simulink model "Model"  (R2020b)
settings: Solver=VariableStepAuto  StartTime=0.0  StopTime=20  MaxStep=0.1  RelTol=1e-1
values from neighbouring files (symbols this model uses):
  D = [0 ... (first row only)    [Data_clean.m]
  g = 9.81    [Data_clean.m]
  k_cart = 0.0113    [Data_clean.m]
  L = 5    [Data_clean.m]
  m = 12000    [Data_clean.m]
  M = 1000    [Data_clean.m]
  Ts = 0.1    [Data_clean.m]
undefined symbols (not defined in the file or in its folder): blk, Discrete, iA, isLTV, lastPcov, lastu, lastx, MDscale, mpc1_plant, MVscale, nCC, nu, nud, nv, nxp, ny, nym, p, RMVscale, Time, ts, uoff, X, xoff, Y, Yscale, Z
libraries: sm_lib x76, mpcsigdimcheck_private x76, nesl_utility x12, ctrlSharedLib x8, simulink_extras x5, mpclib x1
(part 3 of 8)

== system Model/3D3 ==
  X : Inport
  X_dot : Inport  Port=2
  Theta : Inport  Port=3
  Theta_dot : Inport  Port=4
  input2 : Inport  Port=5
  input1 : Inport  Port=6
  Brick Solid : sm_lib/Body Elements/Brick Solid  GraphicAmbientColor=[0.15 0.15 0.15 1.0]  BasedOnType=Mass  BrickDimensions=[15 3 0.5]  BrickDimensionUnits=m  CenterOfMass=[0 0 0]  CenterOfMassUnits=m  GraphicDiffuseColor=[0.5 0.5 0.5]  Density=1000  DensityUnits=kg/m^3  DoExposeReferenceFrame=on  GraphicEmissiveColor=[0.0 0.0 0.0 1.0]  ExportEntireGeometry=off  SerializedFrames=<Frames/>  MarkerShape=Sphere  MarkerSize=10  GraphicType=FromGeometry  InertiaType=CalculateFromGeometry  Mass=12500  MassUnits=kg  MomentsOfInertia=[1 1 1]  MomentsOfInertiaUnits=kg*m^2  GraphicOpacity=1.0  ProductsOfInertia=[0 0 0]  ProductsOfInertiaUnits=kg*m^2  GraphicShininess=75  GraphicSpecularColor=[0.5 0.5 0.5 1.0]  GraphicVisPropType=SimpleVisualProperties
      settings: SourceProductName=Multibody
  Brick Solid1 : sm_lib/Body Elements/Brick Solid  GraphicAmbientColor=[0.15 0.15 0.15 1.0]  BasedOnType=Mass  BrickDimensions=[2 2 0.5]  BrickDimensionUnits=m  CenterOfMass=[0 0 0]  CenterOfMassUnits=m  GraphicDiffuseColor=[1.0 0.2 0.2]  Density=1000  DensityUnits=kg/m^3  DoExposeReferenceFrame=on  GraphicEmissiveColor=[0.0 0.0 0.0 1.0]  ExportEntireGeometry=off  SerializedFrames=<Frames/>  MarkerShape=Sphere  MarkerSize=10  GraphicType=FromGeometry  InertiaType=CalculateFromGeometry  Mass=12500  MassUnits=kg  MomentsOfInertia=[1 1 1]  MomentsOfInertiaUnits=kg*m^2  GraphicOpacity=1.0  ProductsOfInertia=[0 0 0]  ProductsOfInertiaUnits=kg*m^2  GraphicShininess=75  GraphicSpecularColor=[0.5 0.5 0.5 1.0]  GraphicVisPropType=SimpleVisualProperties
      settings: SourceProductName=Multibody
  Cylindrical Solid : sm_lib/Body Elements/Cylindrical Solid  GraphicAmbientColor=[0.15 0.15 0.15 1.0]  BasedOnType=Density  CenterOfMass=[0 0 0]  CenterOfMassUnits=m  GraphicDiffuseColor=[1.0 0.8 0.0]  CylinderLength=L  CylinderLengthUnits=m  CylinderRadius=0.05  CylinderRadiusUnits=m  Density=1000  DensityUnits=kg/m^3  DoExposeReferenceFrame=on  GraphicEmissiveColor=[0.0 0.0 0.0 1.0]  ExportEntireGeometry=off  SerializedFrames=<Frames/>  MarkerShape=Sphere  MarkerSize=10  GraphicType=FromGeometry  InertiaType=CalculateFromGeometry  Mass=1  MassUnits=kg  MomentsOfInertia=[1 1 1]  MomentsOfInertiaUnits=kg*m^2  GraphicOpacity=1.0  ProductsOfInertia=[0 0 0]  ProductsOfInertiaUnits=kg*m^2  GraphicShininess=75  GraphicSpecularColor=[0.5 0.5 0.5 1.0]  GraphicVisPropType=SimpleVisualProperties
  Graphic : sm_lib/Body Elements/Graphic  Commented=on  GraphicType=Marker  MarkerShape=Frame  MarkerSize=20  GraphicVisPropType=SimpleVisualProperties  GraphicDiffuseColor=[0.6 0.6 1.0]  GraphicSpecularColor=[0.5 0.5 0.5 1.0]  GraphicAmbientColor=[0.15 0.15 0.15 1.0]  GraphicEmissiveColor=[0.0 0.0 0.0 1.0]  GraphicShininess=75  GraphicOpacity=1.0
  Graphic1 : sm_lib/Body Elements/Graphic  Commented=on  GraphicType=Marker  MarkerShape=Frame  MarkerSize=20  GraphicVisPropType=SimpleVisualProperties  GraphicDiffuseColor=[1.0 0.2 0.2]  GraphicSpecularColor=[0.5 0.5 0.5 1.0]  GraphicAmbientColor=[0.15 0.15 0.15 1.0]  GraphicEmissiveColor=[0.0 0.0 0.0 1.0]  GraphicShininess=75  GraphicOpacity=1.0
  Graphic2 : sm_lib/Body Elements/Graphic  Commented=on  GraphicType=Marker  MarkerShape=Frame  MarkerSize=20  GraphicVisPropType=SimpleVisualProperties  GraphicDiffuseColor=[0.8 0.8 0.0]  GraphicSpecularColor=[0.5 0.5 0.5 1.0]  GraphicAmbientColor=[0.15 0.15 0.15 1.0]  GraphicEmissiveColor=[0.0 0.0 0.0 1.0]  GraphicShininess=75  GraphicOpacity=1.0
  Graphic3 : sm_lib/Body Elements/Graphic  Commented=on  GraphicType=Marker  MarkerShape=Frame  MarkerSize=20  GraphicVisPropType=SimpleVisualProperties  GraphicDiffuseColor=[0.2 0.2 1.0]  GraphicSpecularColor=[0.5 0.5 0.5 1.0]  GraphicAmbientColor=[0.15 0.15 0.15 1.0]  GraphicEmissiveColor=[0.0 0.0 0.0 1.0]  GraphicShininess=75  GraphicOpacity=1.0
  Graphic4 : sm_lib/Body Elements/Graphic  Commented=on  GraphicType=Marker  MarkerShape=Frame  MarkerSize=20  GraphicVisPropType=SimpleVisualProperties  GraphicDiffuseColor=[0.8 1.0 0.0]  GraphicSpecularColor=[0.5 0.5 0.5 1.0]  GraphicAmbientColor=[0.15 0.15 0.15 1.0]  GraphicEmissiveColor=[0.0 0.0 0.0 1.0]  GraphicShininess=75  GraphicOpacity=1.0
  Mechanism Configuration : sm_lib/Utilities/Mechanism Configuration  UniformGravity=Constant  GravityVector=[0 0 -9.80665]  GravityVectorUnits=m/s^2  GravityUnits=m/s^2  LinearizationDelta=0.001  JointModeTransitionNonlinearIterations=2
      settings: SourceProductName=Multibody
  Prismatic Joint : sm_lib/Joints/Prismatic Joint  JointMode=Normal  SenseConstraintForce=off  SenseConstraintForceX=off  SenseConstraintForceY=off  SenseConstraintForceZ=off  SenseConstraintTorque=off  SenseConstraintTorqueX=off  SenseConstraintTorqueY=off  SenseConstraintTorqueZ=off  SenseTotalForce=off  SenseTotalForceX=off  SenseTotalForceY=off  SenseTotalForceZ=off  SenseTotalTorque=off  SenseTotalTorqueX=off  SenseTotalTorqueY=off  SenseTotalTorqueZ=off  CompositeWrenchDir=FollowerOnBase  CompositeWrenchFrame=BaseFrame  EquilibriumPosition=0  EquilibriumPositionUnits=m  SpringStiffness=0  SpringStiffnessUnits=N/m  DampingCoefficient=0  DampingCoefficientUnits=N/(m/s)  TorqueActuationMode=ComputedTorque  MotionActuationMode=InputMotion  SensePosition=off  SenseVelocity=off  SenseAcceleration=off  SenseTorqueForce=off  SenseLowerLimitTorqueForce=off  SenseUpperLimitTorqueForce=off  LowerLimitSpecify=off  LowerLimitBound=-1  LowerLimitBoundUnits=m  LowerLimitStiffness=1e6  LowerLimitStiffnessUnits=N/m  LowerLimitDamping=1e3  LowerLimitDampingUnits=N/(m/s)  LowerLimitTransitionRegionWidth=1e-4  LowerLimitTransitionRegionWidthUnits=m  UpperLimitSpecify=off  UpperLimitBound=1  UpperLimitBoundUnits=m  UpperLimitStiffness=1e6  UpperLimitStiffnessUnits=N/m  UpperLimitDamping=1e3  UpperLimitDampingUnits=N/(m/s)  UpperLimitTransitionRegionWidth=1e-4  UpperLimitTransitionRegionWidthUnits=m  PositionTargetSpecify=off  PositionTargetPriority=High  PositionTargetValue=0  PositionTargetValueUnits=m  VelocityTargetSpecify=off  VelocityTargetPriority=High  VelocityTargetValue=0  VelocityTargetValueUnits=m/s
  Revolute Joint : sm_lib/Joints/Revolute Joint  JointMode=Normal  SenseConstraintForce=off  SenseConstraintForceX=off  SenseConstraintForceY=off  SenseConstraintForceZ=off  SenseConstraintTorque=off  SenseConstraintTorqueX=off  SenseConstraintTorqueY=off  SenseConstraintTorqueZ=off  SenseTotalForce=off  SenseTotalForceX=off  SenseTotalForceY=off  SenseTotalForceZ=off  SenseTotalTorque=off  SenseTotalTorqueX=off  SenseTotalTorqueY=off  SenseTotalTorqueZ=off  CompositeWrenchDir=FollowerOnBase  CompositeWrenchFrame=BaseFrame  EquilibriumPosition=0  EquilibriumPositionUnits=deg  SpringStiffness=0  SpringStiffnessUnits=N*m/deg  DampingCoefficient=0  DampingCoefficientUnits=N*m/(deg/s)  TorqueActuationMode=ComputedTorque  MotionActuationMode=InputMotion  SensePosition=off  SenseVelocity=off  SenseAcceleration=off  SenseTorqueForce=off  SenseLowerLimitTorqueForce=off  SenseUpperLimitTorqueForce=off  LowerLimitSpecify=off  LowerLimitBound=-90  LowerLimitBoundUnits=deg  LowerLimitStiffness=1e4  LowerLimitStiffnessUnits=N*m/deg  LowerLimitDamping=10  LowerLimitDampingUnits=N*m/(deg/s)  LowerLimitTransitionRegionWidth=0.1  LowerLimitTransitionRegionWidthUnits=deg  UpperLimitSpecify=off  UpperLimitBound=90  UpperLimitBoundUnits=deg  UpperLimitStiffness=1e4  UpperLimitStiffnessUnits=N*m/deg  UpperLimitDamping=10  UpperLimitDampingUnits=N*m/(deg/s)  UpperLimitTransitionRegionWidth=0.1  UpperLimitTransitionRegionWidthUnits=deg  PositionTargetSpecify=off  PositionTargetPriority=High  PositionTargetValue=0.2  PositionTargetValueUnits=rad  VelocityTargetSpecify=off  VelocityTargetPriority=High  VelocityTargetValue=0  VelocityTargetValueUnits=deg/s
  Rigid Transform : sm_lib/Frames and Transforms/Rigid Transform  TranslationMethod=StandardAxis  TranslationStandardOffset=6.5  TranslationLengthUnit=m  TranslationStandardAxis=-X  TranslationCartesianOffset=[0 0 0]  TranslationROffset=0  TranslationROffsetUnits=m  TranslationZOffset=0  TranslationZOffsetUnits=m  TranslationThetaOffset=0  TranslationThetaOffsetUnits=deg  RotationMethod=None  RotationAngleUnits=deg  RotationStandardAxis=+Z  RotationAngle=0.0  RotationArbitraryAxis=[0 0 1]  FollAlignAxisA=+X  BaseAlignAxisA=+X  FollAlignAxisB=+Z  BaseAlignAxisB=-Z  RotationSequenceAxes=FollowerAxes  RotationSequence=XYX  RotationSequenceAngles=[0 0 0]  RotationSequenceAnglesUnits=deg  RotationMatrix=[1 0 0; 0 1 0; 0 0 1]
      settings: SourceProductName=Multibody
  Rigid Transform1 : sm_lib/Frames and Transforms/Rigid Transform  TranslationMethod=None  TranslationStandardOffset=0.5  TranslationLengthUnit=m  TranslationStandardAxis=+Z  TranslationCartesianOffset=[0 0 0]  TranslationROffset=0  TranslationROffsetUnits=m  TranslationZOffset=0  TranslationZOffsetUnits=m  TranslationThetaOffset=0  TranslationThetaOffsetUnits=deg  RotationMethod=AlignedAxes  RotationAngleUnits=deg  RotationStandardAxis=+Z  RotationAngle=0.0  RotationArbitraryAxis=[0 0 1]  FollAlignAxisA=+X  BaseAlignAxisA=+Z  FollAlignAxisB=+Y  BaseAlignAxisB=+Y  RotationSequenceAxes=FollowerAxes  RotationSequence=XYX  RotationSequenceAngles=[0 0 0]  RotationSequenceAnglesUnits=deg  RotationMatrix=[1 0 0; 0 1 0; 0 0 1]
      settings: SourceProductName=Multibody
  Rigid Transform2 : sm_lib/Frames and Transforms/Rigid Transform  TranslationMethod=StandardAxis  TranslationStandardOffset=0.5  TranslationLengthUnit=m  TranslationStandardAxis=+Z  TranslationCartesianOffset=[0 0 0]  TranslationROffset=0  TranslationROffsetUnits=m  TranslationZOffset=0  TranslationZOffsetUnits=m  TranslationThetaOffset=0  TranslationThetaOffsetUnits=deg  RotationMethod=AlignedAxes  RotationAngleUnits=deg  RotationStandardAxis=+Z  RotationAngle=0.0  RotationArbitraryAxis=[0 0 1]  FollAlignAxisA=+Z  BaseAlignAxisA=+X  FollAlignAxisB=+Y  BaseAlignAxisB=+Y  RotationSequenceAxes=FollowerAxes  RotationSequence=XYX  RotationSequenceAngles=[0 0 0]  RotationSequenceAnglesUnits=deg  RotationMatrix=[1 0 0; 0 1 0; 0 0 1]
      settings: SourceProductName=Multibody
  Rigid Transform3 : sm_lib/Frames and Transforms/Rigid Transform  TranslationMethod=StandardAxis  TranslationStandardOffset=L/2  TranslationLengthUnit=m  TranslationStandardAxis=-Z  TranslationCartesianOffset=[0 0 0]  TranslationROffset=0  TranslationROffsetUnits=m  TranslationZOffset=0  TranslationZOffsetUnits=m  TranslationThetaOffset=0  TranslationThetaOffsetUnits=deg  RotationMethod=None  RotationAngleUnits=deg  RotationStandardAxis=+Z  RotationAngle=0.0  RotationArbitraryAxis=[0 0 1]  FollAlignAxisA=+X  BaseAlignAxisA=+X  FollAlignAxisB=+Z  BaseAlignAxisB=+Y  RotationSequenceAxes=FollowerAxes  RotationSequence=XYX  RotationSequenceAngles=[0 0 0]  RotationSequenceAnglesUnits=deg  RotationMatrix=[1 0 0; 0 1 0; 0 0 1]
      settings: SourceProductName=Multibody
  Rigid Transform4 : sm_lib/Frames and Transforms/Rigid Transform  TranslationMethod=None  TranslationStandardOffset=2.5  TranslationLengthUnit=m  TranslationStandardAxis=-Z  TranslationCartesianOffset=[0 0 0]  TranslationROffset=0  TranslationROffsetUnits=m  TranslationZOffset=0  TranslationZOffsetUnits=m  TranslationThetaOffset=0  TranslationThetaOffsetUnits=deg  RotationMethod=AlignedAxes  RotationAngleUnits=deg  RotationStandardAxis=+Z  RotationAngle=0.0  RotationArbitraryAxis=[0 0 1]  FollAlignAxisA=+X  BaseAlignAxisA=+X  FollAlignAxisB=+Y  BaseAlignAxisB=+Z  RotationSequenceAxes=FollowerAxes  RotationSequence=XYX  RotationSequenceAngles=[0 0 0]  RotationSequenceAnglesUnits=deg  RotationMatrix=[1 0 0; 0 1 0; 0 0 1]
      settings: SourceProductName=Multibody
  Rigid Transform5 : sm_lib/Frames and Transforms/Rigid Transform  TranslationMethod=StandardAxis  TranslationStandardOffset=L/2  TranslationLengthUnit=m  TranslationStandardAxis=-Y  TranslationCartesianOffset=[0 0 0]  TranslationROffset=0  TranslationROffsetUnits=m  TranslationZOffset=0  TranslationZOffsetUnits=m  TranslationThetaOffset=0  TranslationThetaOffsetUnits=deg  RotationMethod=AlignedAxes  RotationAngleUnits=deg  RotationStandardAxis=+Z  RotationAngle=0.0  RotationArbitraryAxis=[0 0 1]  FollAlignAxisA=+X  BaseAlignAxisA=+X  FollAlignAxisB=+Z  BaseAlignAxisB=+Y  RotationSequenceAxes=FollowerAxes  RotationSequence=XYX  RotationSequenceAngles=[0 0 0]  RotationSequenceAnglesUnits=deg  RotationMatrix=[1 0 0; 0 1 0; 0 0 1]
      settings: SourceProductName=Multibody
  Simulink-PS Converter : nesl_utility/Simulink-PS Converter  PhysicalDomain=network_engine_domain  SubClassName=ps_input  LeftPortType=input  RightPortType=output  PseudoPeriodic=off  Frequencies=[]  NoiseDistribution=none  NoiseParameters=[]  Unit=1  AffineConversion=off  FilteringAndDerivatives=provide  SimscapeFilterOrder=1  InputFilterTimeConstant=0.001  UdotUserProvided=2
  Simulink-PS Converter1 : nesl_utility/Simulink-PS Converter  PhysicalDomain=network_engine_domain  SubClassName=ps_input  LeftPortType=input  RightPortType=output  PseudoPeriodic=off  Frequencies=[]  NoiseDistribution=none  NoiseParameters=[]  Unit=1  AffineConversion=off  FilteringAndDerivatives=provide  SimscapeFilterOrder=1  InputFilterTimeConstant=0.001  UdotUserProvided=2
  Solver Configuration : nesl_utility/Solver Configuration  PhysicalDomain=network_engine_domain  SubClassName=solver  LeftPortType=input  RightPortType=generic  Tones=[]  Harmonics=[]  SimulateNoise=off  Profile=off  UseLocalSampling=off  EnableSwitchedLinearOptims=on  FrequencyDomain=off  UseCCode=off  RelTol=0.001  AbsTol=1e-06  MinStep=1e-09  ToWorkspace=off  RevertToSquareIcSolve=off  NumHomotopyIterations=100  PhasorMode=off  PhasorModeNumHarmonics=1  DoDC=off  ResidualTolerance=1e-09  UseLocalSolver=off  LocalSolverChoice=NE_BACKWARD_EULER_ADVANCER  LocalSolverSampleTime=0.001  DoFixedCost=off  MaxNonlinIter=3  MaxModeIter=2  ComputeImpulses=off  ImpulseIterations=2  LinearAlgebra=Sparse  EquationFormulation=NE_TIME_EF  DelaysMemoryBudget=1024  AutomaticFiltering=on  FilteringTimeConstant=0.001  PartitionStorageMethod=AS_NEEDED  PartitionMemoryBudget=1024  PartitionMethod=FAST
      settings: SourceProductName=Utilities
  Spherical Solid : sm_lib/Body Elements/Spherical Solid  GraphicAmbientColor=[0.15 0.15 0.15 1.0]  BasedOnType=Density  CenterOfMass=[0 0 0]  CenterOfMassUnits=m  GraphicDiffuseColor=[0.2 0.8 0.0]  Density=1000  DensityUnits=kg/m^3  DoExposeReferenceFrame=on  GraphicEmissiveColor=[0.0 0.0 0.0 1.0]  ExportEntireGeometry=off  SerializedExposedGeometries=<ExposedGeometries/>  SerializedFrames=<Frames/>  MarkerShape=Sphere  MarkerSize=10  GraphicType=FromGeometry  InertiaType=CalculateFromGeometry  Mass=1  MassUnits=kg  MomentsOfInertia=[1 1 1]  MomentsOfInertiaUnits=kg*m^2  GraphicOpacity=1.0  ProductsOfInertia=[0 0 0]  ProductsOfInertiaUnits=kg*m^2  GraphicShininess=75  GraphicSpecularColor=[0.5 0.5 0.5 1.0]  SphereRadius=0.5  SphereRadiusUnits=m  GraphicVisPropType=SimpleVisualProperties
  World Frame : sm_lib/Frames and Transforms/World Frame
      settings: SourceProductName=Multibody
  wires:
  Theta_dot/1 -> Simulink-PS Converter1/2
  input2/1 -> Simulink-PS Converter/3
  X/1 -> Simulink-PS Converter/1
  X_dot/1 -> Simulink-PS Converter/2
  Theta/1 -> Simulink-PS Converter1/1
  input1/1 -> Simulink-PS Converter1/3
  connections:
  Rigid Transform5/LConn1 -- Graphic3/RConn1 -- Revolute Joint/RConn1
  Rigid Transform3/LConn1 -- Rigid Transform5/RConn1 -- Cylindrical Solid/RConn1 -- Graphic4/RConn1
  Simulink-PS Converter1/RConn1 -- Revolute Joint/LConn2
  Rigid Transform4/LConn1 -- Brick Solid1/RConn1 -- Graphic2/RConn1 -- Rigid Transform1/RConn1
  Brick Solid/RConn1 -- Graphic/RConn1 -- World Frame/RConn1 -- Mechanism Configuration/RConn1 -- Solver Configuration/RConn1 -- Rigid Transform/LConn1
  Simulink-PS Converter/RConn1 -- Prismatic Joint/LConn2
  Rigid Transform1/LConn1 -- Prismatic Joint/RConn1
  Prismatic Joint/LConn1 -- Graphic1/RConn1 -- Rigid Transform2/RConn1
  Rigid Transform3/RConn1 -- Spherical Solid/RConn1
  Rigid Transform2/LConn1 -- Rigid Transform/RConn1
  Revolute Joint/LConn1 -- Rigid Transform4/RConn1

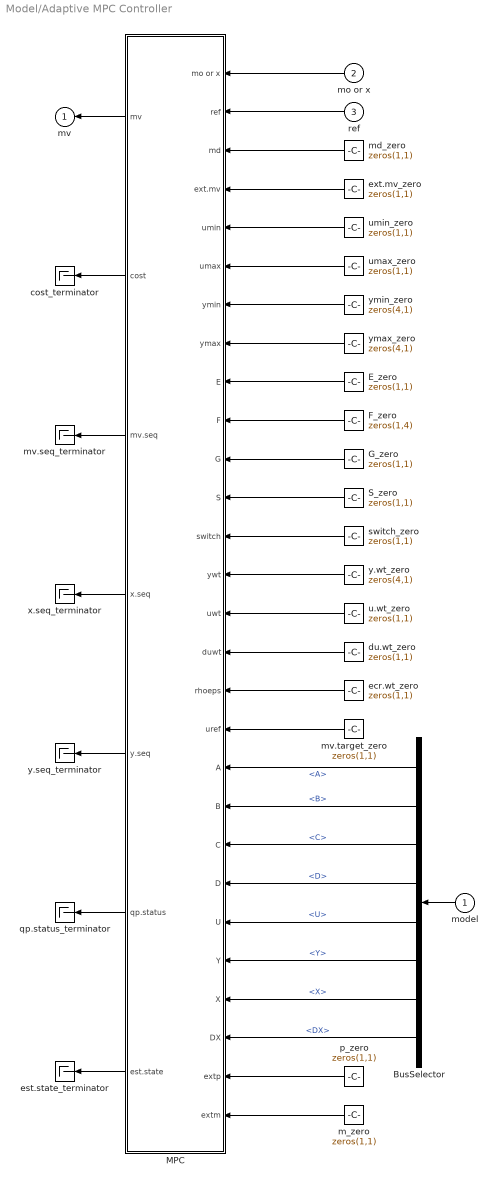
== system Model/Adaptive MPC Controller ==
  model : Inport
  mo or x : Inport  Port=2
  ref : Inport  Port=3
  BusSelector : BusSelector  OutputSignals=A,B,C,D,U,Y,X,DX
  E_zero : Constant  Value=zeros(1,1)  VectorParams1D=off  OutDataTypeStr=BlockDataType
  F_zero : Constant  Value=zeros(1,4)  VectorParams1D=off  OutDataTypeStr=BlockDataType
  G_zero : Constant  Value=zeros(1,1)  VectorParams1D=off  OutDataTypeStr=BlockDataType
  MPC : Subsystem
  S_zero : Constant  Value=zeros(1,1)  VectorParams1D=off  OutDataTypeStr=BlockDataType
  cost_terminator : Terminator
  du.wt_zero : Constant  Value=zeros(1,1)  OutDataTypeStr=BlockDataType
  ecr.wt_zero : Constant  Value=zeros(1,1)  OutDataTypeStr=BlockDataType
  est.state_terminator : Terminator
  ext.mv_zero : Constant  Value=zeros(1,1)  OutDataTypeStr=BlockDataType
  m_zero : Constant  Value=zeros(1,1)  OutDataTypeStr=BlockDataType
  md_zero : Constant  Value=zeros(1,1)  OutDataTypeStr=BlockDataType
  mv.seq_terminator : Terminator
  mv.target_zero : Constant  Value=zeros(1,1)  OutDataTypeStr=BlockDataType
  p_zero : Constant  Value=zeros(1,1)  OutDataTypeStr=BlockDataType
  qp.status_terminator : Terminator
  switch_zero : Constant  Value=zeros(1,1)  OutDataTypeStr=BlockDataType
  u.wt_zero : Constant  Value=zeros(1,1)  OutDataTypeStr=BlockDataType
  umax_zero : Constant  Value=zeros(1,1)  OutDataTypeStr=BlockDataType
  umin_zero : Constant  Value=zeros(1,1)  OutDataTypeStr=BlockDataType
  x.seq_terminator : Terminator
  y.seq_terminator : Terminator
  y.wt_zero : Constant  Value=zeros(4,1)  OutDataTypeStr=BlockDataType
  ymax_zero : Constant  Value=zeros(4,1)  OutDataTypeStr=BlockDataType
  ymin_zero : Constant  Value=zeros(4,1)  OutDataTypeStr=BlockDataType
  mv : Outport  VectorParamsAs1DForOutWhenUnconnected=off
  wires:
  m_zero/1 -> MPC/28(extm)
  p_zero/1 -> MPC/27(extp)
  MPC/5(y.seq) -> y.seq_terminator/1
  MPC/4(x.seq) -> x.seq_terminator/1
  G_zero/1 -> MPC/11(G)
  F_zero/1 -> MPC/10(F)
  E_zero/1 -> MPC/9(E)
  S_zero/1 -> MPC/12(S)
  MPC/7(est.state) -> est.state_terminator/1
  y.wt_zero/1 -> MPC/14(ywt)
  switch_zero/1 -> MPC/13(switch)
  ymin_zero/1 -> MPC/7(ymin)
  umax_zero/1 -> MPC/6(umax)
  umin_zero/1 -> MPC/5(umin)
  u.wt_zero/1 -> MPC/15(uwt)
  ymax_zero/1 -> MPC/8(ymax)
  du.wt_zero/1 -> MPC/16(duwt)
  ecr.wt_zero/1 -> MPC/17(rhoeps)
  mv.target_zero/1 -> MPC/18(uref)
  ext.mv_zero/1 -> MPC/4(ext.mv)
  BusSelector/8 -> MPC/26(DX)  "<DX>"
  BusSelector/5 -> MPC/23(U)  "<U>"
  model/1 -> BusSelector/1
  BusSelector/4 -> MPC/22(D)  "<D>"
  BusSelector/3 -> MPC/21(C)  "<C>"
  BusSelector/2 -> MPC/20(B)  "<B>"
  BusSelector/1 -> MPC/19(A)  "<A>"
  MPC/6(qp.status) -> qp.status_terminator/1
  MPC/3(mv.seq) -> mv.seq_terminator/1
  MPC/2(cost) -> cost_terminator/1
  ref/1 -> MPC/2(ref)
  mo or x/1 -> MPC/1(mo or x)
  MPC/1(mv) -> mv/1
  md_zero/1 -> MPC/3(md)
  BusSelector/7 -> MPC/25(X)  "<X>"
  BusSelector/6 -> MPC/24(Y)  "<Y>"

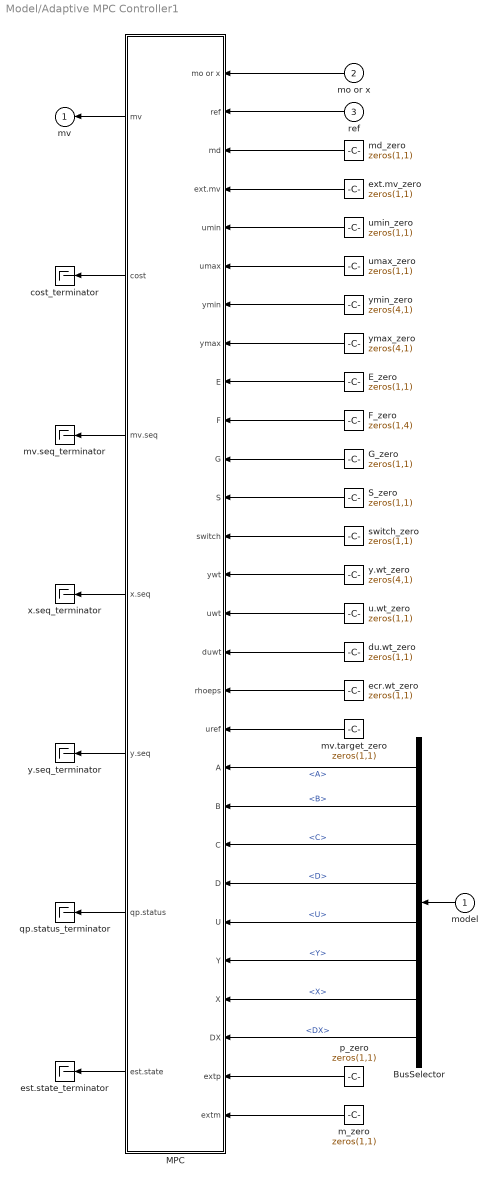
== system Model/Adaptive MPC Controller1 ==
  model : Inport
  mo or x : Inport  Port=2
  ref : Inport  Port=3
  BusSelector : BusSelector  OutputSignals=A,B,C,D,U,Y,X,DX
  E_zero : Constant  Value=zeros(1,1)  VectorParams1D=off  OutDataTypeStr=BlockDataType
  F_zero : Constant  Value=zeros(1,4)  VectorParams1D=off  OutDataTypeStr=BlockDataType
  G_zero : Constant  Value=zeros(1,1)  VectorParams1D=off  OutDataTypeStr=BlockDataType
  MPC : Subsystem
  S_zero : Constant  Value=zeros(1,1)  VectorParams1D=off  OutDataTypeStr=BlockDataType
  cost_terminator : Terminator
  du.wt_zero : Constant  Value=zeros(1,1)  OutDataTypeStr=BlockDataType
  ecr.wt_zero : Constant  Value=zeros(1,1)  OutDataTypeStr=BlockDataType
  est.state_terminator : Terminator
  ext.mv_zero : Constant  Value=zeros(1,1)  OutDataTypeStr=BlockDataType
  m_zero : Constant  Value=zeros(1,1)  OutDataTypeStr=BlockDataType
  md_zero : Constant  Value=zeros(1,1)  OutDataTypeStr=BlockDataType
  mv.seq_terminator : Terminator
  mv.target_zero : Constant  Value=zeros(1,1)  OutDataTypeStr=BlockDataType
  p_zero : Constant  Value=zeros(1,1)  OutDataTypeStr=BlockDataType
  qp.status_terminator : Terminator
  switch_zero : Constant  Value=zeros(1,1)  OutDataTypeStr=BlockDataType
  u.wt_zero : Constant  Value=zeros(1,1)  OutDataTypeStr=BlockDataType
  umax_zero : Constant  Value=zeros(1,1)  OutDataTypeStr=BlockDataType
  umin_zero : Constant  Value=zeros(1,1)  OutDataTypeStr=BlockDataType
  x.seq_terminator : Terminator
  y.seq_terminator : Terminator
  y.wt_zero : Constant  Value=zeros(4,1)  OutDataTypeStr=BlockDataType
  ymax_zero : Constant  Value=zeros(4,1)  OutDataTypeStr=BlockDataType
  ymin_zero : Constant  Value=zeros(4,1)  OutDataTypeStr=BlockDataType
  mv : Outport  VectorParamsAs1DForOutWhenUnconnected=off
  wires:
  m_zero/1 -> MPC/28(extm)
  p_zero/1 -> MPC/27(extp)
  MPC/5(y.seq) -> y.seq_terminator/1
  MPC/4(x.seq) -> x.seq_terminator/1
  G_zero/1 -> MPC/11(G)
  F_zero/1 -> MPC/10(F)
  E_zero/1 -> MPC/9(E)
  S_zero/1 -> MPC/12(S)
  MPC/7(est.state) -> est.state_terminator/1
  y.wt_zero/1 -> MPC/14(ywt)
  switch_zero/1 -> MPC/13(switch)
  ymin_zero/1 -> MPC/7(ymin)
  umax_zero/1 -> MPC/6(umax)
  umin_zero/1 -> MPC/5(umin)
  u.wt_zero/1 -> MPC/15(uwt)
  ymax_zero/1 -> MPC/8(ymax)
  du.wt_zero/1 -> MPC/16(duwt)
  ecr.wt_zero/1 -> MPC/17(rhoeps)
  mv.target_zero/1 -> MPC/18(uref)
  ext.mv_zero/1 -> MPC/4(ext.mv)
  BusSelector/8 -> MPC/26(DX)  "<DX>"
  BusSelector/5 -> MPC/23(U)  "<U>"
  model/1 -> BusSelector/1
  BusSelector/4 -> MPC/22(D)  "<D>"
  BusSelector/3 -> MPC/21(C)  "<C>"
  BusSelector/2 -> MPC/20(B)  "<B>"
  BusSelector/1 -> MPC/19(A)  "<A>"
  MPC/6(qp.status) -> qp.status_terminator/1
  MPC/3(mv.seq) -> mv.seq_terminator/1
  MPC/2(cost) -> cost_terminator/1
  ref/1 -> MPC/2(ref)
  mo or x/1 -> MPC/1(mo or x)
  MPC/1(mv) -> mv/1
  md_zero/1 -> MPC/3(md)
  BusSelector/7 -> MPC/25(X)  "<X>"
  BusSelector/6 -> MPC/24(Y)  "<Y>"

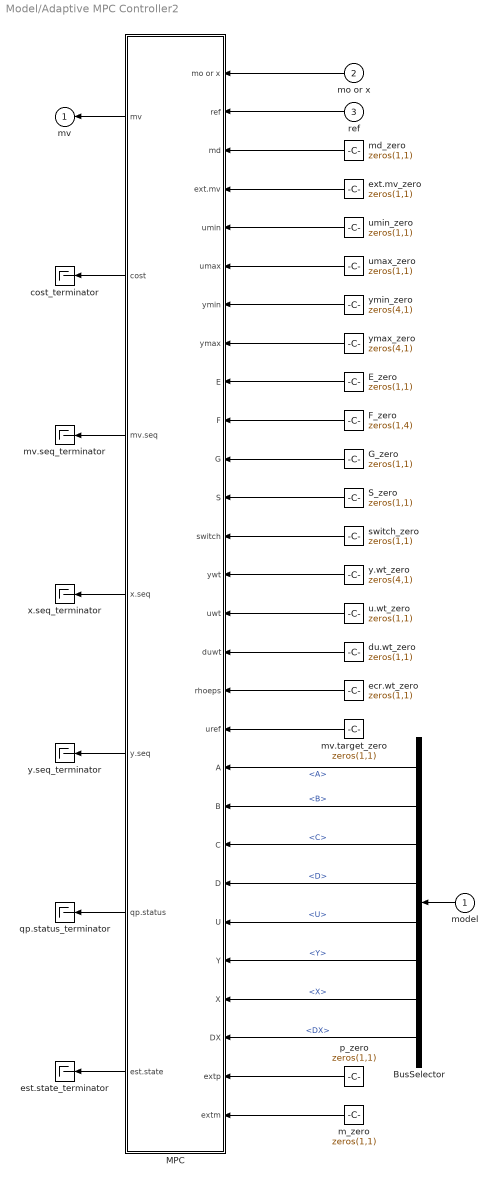
== system Model/Adaptive MPC Controller2 ==
  model : Inport
  mo or x : Inport  Port=2
  ref : Inport  Port=3
  BusSelector : BusSelector  OutputSignals=A,B,C,D,U,Y,X,DX
  E_zero : Constant  Value=zeros(1,1)  VectorParams1D=off  OutDataTypeStr=BlockDataType
  F_zero : Constant  Value=zeros(1,4)  VectorParams1D=off  OutDataTypeStr=BlockDataType
  G_zero : Constant  Value=zeros(1,1)  VectorParams1D=off  OutDataTypeStr=BlockDataType
  MPC : Subsystem
  S_zero : Constant  Value=zeros(1,1)  VectorParams1D=off  OutDataTypeStr=BlockDataType
  cost_terminator : Terminator
  du.wt_zero : Constant  Value=zeros(1,1)  OutDataTypeStr=BlockDataType
  ecr.wt_zero : Constant  Value=zeros(1,1)  OutDataTypeStr=BlockDataType
  est.state_terminator : Terminator
  ext.mv_zero : Constant  Value=zeros(1,1)  OutDataTypeStr=BlockDataType
  m_zero : Constant  Value=zeros(1,1)  OutDataTypeStr=BlockDataType
  md_zero : Constant  Value=zeros(1,1)  OutDataTypeStr=BlockDataType
  mv.seq_terminator : Terminator
  mv.target_zero : Constant  Value=zeros(1,1)  OutDataTypeStr=BlockDataType
  p_zero : Constant  Value=zeros(1,1)  OutDataTypeStr=BlockDataType
  qp.status_terminator : Terminator
  switch_zero : Constant  Value=zeros(1,1)  OutDataTypeStr=BlockDataType
  u.wt_zero : Constant  Value=zeros(1,1)  OutDataTypeStr=BlockDataType
  umax_zero : Constant  Value=zeros(1,1)  OutDataTypeStr=BlockDataType
  umin_zero : Constant  Value=zeros(1,1)  OutDataTypeStr=BlockDataType
  x.seq_terminator : Terminator
  y.seq_terminator : Terminator
  y.wt_zero : Constant  Value=zeros(4,1)  OutDataTypeStr=BlockDataType
  ymax_zero : Constant  Value=zeros(4,1)  OutDataTypeStr=BlockDataType
  ymin_zero : Constant  Value=zeros(4,1)  OutDataTypeStr=BlockDataType
  mv : Outport  VectorParamsAs1DForOutWhenUnconnected=off
  wires:
  m_zero/1 -> MPC/28(extm)
  p_zero/1 -> MPC/27(extp)
  MPC/5(y.seq) -> y.seq_terminator/1
  MPC/4(x.seq) -> x.seq_terminator/1
  G_zero/1 -> MPC/11(G)
  F_zero/1 -> MPC/10(F)
  E_zero/1 -> MPC/9(E)
  S_zero/1 -> MPC/12(S)
  MPC/7(est.state) -> est.state_terminator/1
  y.wt_zero/1 -> MPC/14(ywt)
  switch_zero/1 -> MPC/13(switch)
  ymin_zero/1 -> MPC/7(ymin)
  umax_zero/1 -> MPC/6(umax)
  umin_zero/1 -> MPC/5(umin)
  u.wt_zero/1 -> MPC/15(uwt)
  ymax_zero/1 -> MPC/8(ymax)
  du.wt_zero/1 -> MPC/16(duwt)
  ecr.wt_zero/1 -> MPC/17(rhoeps)
  mv.target_zero/1 -> MPC/18(uref)
  ext.mv_zero/1 -> MPC/4(ext.mv)
  BusSelector/8 -> MPC/26(DX)  "<DX>"
  BusSelector/5 -> MPC/23(U)  "<U>"
  model/1 -> BusSelector/1
  BusSelector/4 -> MPC/22(D)  "<D>"
  BusSelector/3 -> MPC/21(C)  "<C>"
  BusSelector/2 -> MPC/20(B)  "<B>"
  BusSelector/1 -> MPC/19(A)  "<A>"
  MPC/6(qp.status) -> qp.status_terminator/1
  MPC/3(mv.seq) -> mv.seq_terminator/1
  MPC/2(cost) -> cost_terminator/1
  ref/1 -> MPC/2(ref)
  mo or x/1 -> MPC/1(mo or x)
  MPC/1(mv) -> mv/1
  md_zero/1 -> MPC/3(md)
  BusSelector/7 -> MPC/25(X)  "<X>"
  BusSelector/6 -> MPC/24(Y)  "<Y>"

== system Model/Adaptive MPC Controller3 ==
  model : Inport
  mo or x : Inport  Port=2
  ref : Inport  Port=3
  BusSelector : BusSelector  OutputSignals=A,B,C,D,U,Y,X,DX
  E_zero : Constant  Value=zeros(1,1)  VectorParams1D=off  OutDataTypeStr=BlockDataType
  F_zero : Constant  Value=zeros(1,4)  VectorParams1D=off  OutDataTypeStr=BlockDataType
  G_zero : Constant  Value=zeros(1,1)  VectorParams1D=off  OutDataTypeStr=BlockDataType
  MPC : Subsystem
  S_zero : Constant  Value=zeros(1,1)  VectorParams1D=off  OutDataTypeStr=BlockDataType
  cost_terminator : Terminator
  du.wt_zero : Constant  Value=zeros(1,1)  OutDataTypeStr=BlockDataType
  ecr.wt_zero : Constant  Value=zeros(1,1)  OutDataTypeStr=BlockDataType
  est.state_terminator : Terminator
  ext.mv_zero : Constant  Value=zeros(1,1)  OutDataTypeStr=BlockDataType
  m_zero : Constant  Value=zeros(1,1)  OutDataTypeStr=BlockDataType
  md_zero : Constant  Value=zeros(1,1)  OutDataTypeStr=BlockDataType
  mv.seq_terminator : Terminator
  mv.target_zero : Constant  Value=zeros(1,1)  OutDataTypeStr=BlockDataType
  p_zero : Constant  Value=zeros(1,1)  OutDataTypeStr=BlockDataType
  qp.status_terminator : Terminator
  switch_zero : Constant  Value=zeros(1,1)  OutDataTypeStr=BlockDataType
  u.wt_zero : Constant  Value=zeros(1,1)  OutDataTypeStr=BlockDataType
  umax_zero : Constant  Value=zeros(1,1)  OutDataTypeStr=BlockDataType
  umin_zero : Constant  Value=zeros(1,1)  OutDataTypeStr=BlockDataType
  x.seq_terminator : Terminator
  y.seq_terminator : Terminator
  y.wt_zero : Constant  Value=zeros(4,1)  OutDataTypeStr=BlockDataType
  ymax_zero : Constant  Value=zeros(4,1)  OutDataTypeStr=BlockDataType
  ymin_zero : Constant  Value=zeros(4,1)  OutDataTypeStr=BlockDataType
  mv : Outport  VectorParamsAs1DForOutWhenUnconnected=off
  wires:
  m_zero/1 -> MPC/28(extm)
  p_zero/1 -> MPC/27(extp)
  MPC/5(y.seq) -> y.seq_terminator/1
  MPC/4(x.seq) -> x.seq_terminator/1
  G_zero/1 -> MPC/11(G)
  F_zero/1 -> MPC/10(F)
  E_zero/1 -> MPC/9(E)
  S_zero/1 -> MPC/12(S)
  MPC/7(est.state) -> est.state_terminator/1
  y.wt_zero/1 -> MPC/14(ywt)
  switch_zero/1 -> MPC/13(switch)
  ymin_zero/1 -> MPC/7(ymin)
  umax_zero/1 -> MPC/6(umax)
  umin_zero/1 -> MPC/5(umin)
  u.wt_zero/1 -> MPC/15(uwt)
  ymax_zero/1 -> MPC/8(ymax)
  du.wt_zero/1 -> MPC/16(duwt)
  ecr.wt_zero/1 -> MPC/17(rhoeps)
  mv.target_zero/1 -> MPC/18(uref)
  ext.mv_zero/1 -> MPC/4(ext.mv)
  BusSelector/8 -> MPC/26(DX)  "<DX>"
  BusSelector/5 -> MPC/23(U)  "<U>"
  model/1 -> BusSelector/1
  BusSelector/4 -> MPC/22(D)  "<D>"
  BusSelector/3 -> MPC/21(C)  "<C>"
  BusSelector/2 -> MPC/20(B)  "<B>"
  BusSelector/1 -> MPC/19(A)  "<A>"
  MPC/6(qp.status) -> qp.status_terminator/1
  MPC/3(mv.seq) -> mv.seq_terminator/1
  MPC/2(cost) -> cost_terminator/1
  ref/1 -> MPC/2(ref)
  mo or x/1 -> MPC/1(mo or x)
  MPC/1(mv) -> mv/1
  md_zero/1 -> MPC/3(md)
  BusSelector/7 -> MPC/25(X)  "<X>"
  BusSelector/6 -> MPC/24(Y)  "<Y>"

== system Model/Crane ==
  note: Rolling Resistance Model
  f : Inport
  Add2 : Sum  Inputs=+-+-
  Add3 : Sum  Inputs=--
  Cos : Trigonometry  Operator=cos
  Gain10 : Gain  Gain=m*g*L
  Gain2 : Gain  Gain=(m+M)*g*k_cart
  Gain5 : Gain  Gain=1/(m*L^2)
  Gain6 : Gain  Gain=1/(M + m)
  Gain7 : Gain  Gain=m*L
  Gain8 : Gain  Gain=m*L
  Gain9 : Gain  Gain=m*L
  Product : Product
  Product1 : Product
  Product2 : Product
  Sin : Trigonometry
  Square : Math  Operator=square  SaturateOnIntegerOverflow=on
  Theta : Integrator
  Theta_dot : Integrator
  X : Integrator
  X_dot : Integrator
  x : Outport
  x_dot : Outport  Port=2
  theta : Outport  Port=3
  theta_dot : Outport  Port=4
  wires:
  Gain5/1 -> Product/2, Theta_dot/1  "Theta_2dot"
  Gain9/1 -> Add3/1  "m * l * x_2dot*cos(Theta)"
  Add3/1 -> Gain5/1
  Product/1 -> Gain7/1  "Theta_2dot*cos(Thetta)"
  Cos/1 -> Product/1, Product2/2  "cos(Theta)"
  Theta_dot/1 -> theta_dot/1, Square/1, Theta/1  "Theta_dot"
  Sin/1 -> Gain10/1, Product1/1  "sin(Theta)"
  Theta/1 -> theta/1, Cos/1, Sin/1  "Theta"
  Gain10/1 -> Add3/2  "m * g * l * sin(Theta)"
  Product2/1 -> Gain9/1  "x_2dot*cos(Theta)"
  Square/1 -> Product1/2  "Thetta_dot^2"
  Gain8/1 -> Add2/3  "m * l * Thetta_dot^2 * sin(Thetta)"
  Gain6/1 -> Product2/1, X_dot/1  "x_2dot"
  X/1 -> x/1  "x"
  X_dot/1 -> x_dot/1, Gain2/1, X/1  "x_dot"
  Gain7/1 -> Add2/2  "m * l * Thetta_2dot * cos(Thetta)"
  Product1/1 -> Gain8/1  "Theta_dot^2 * sin(Theta)"
  f/1 -> Add2/1
  Add2/1 -> Gain6/1
  Gain2/1 -> Add2/4

== system Model/Crane 1 ==
  note: Rolling Resistance Model
  f : Inport
  Add2 : Sum  Inputs=+-+-
  Add3 : Sum  Inputs=--
  Cos : Trigonometry  Operator=cos
  Gain10 : Gain  Gain=m*g*L
  Gain2 : Gain  Gain=(m+M)*g*k_cart
  Gain5 : Gain  Gain=1/(m*L^2)
  Gain6 : Gain  Gain=1/(M + m)
  Gain7 : Gain  Gain=m*L
  Gain8 : Gain  Gain=m*L
  Gain9 : Gain  Gain=m*L
  Product : Product
  Product1 : Product
  Product2 : Product
  Sin : Trigonometry
  Square : Math  Operator=square  SaturateOnIntegerOverflow=on
  Theta : Integrator
  Theta_dot : Integrator
  X : Integrator
  X_dot : Integrator
  x : Outport
  x_dot : Outport  Port=2
  theta : Outport  Port=3
  theta_dot : Outport  Port=4
  wires:
  Gain5/1 -> Product/2, Theta_dot/1  "Theta_2dot"
  Gain9/1 -> Add3/1  "m * l * x_2dot*cos(Theta)"
  Add3/1 -> Gain5/1
  Product/1 -> Gain7/1  "Theta_2dot*cos(Thetta)"
  Cos/1 -> Product/1, Product2/2  "cos(Theta)"
  Theta_dot/1 -> theta_dot/1, Square/1, Theta/1  "Theta_dot"
  Sin/1 -> Gain10/1, Product1/1  "sin(Theta)"
  Theta/1 -> theta/1, Cos/1, Sin/1  "Theta"
  Gain10/1 -> Add3/2  "m * g * l * sin(Theta)"
  Product2/1 -> Gain9/1  "x_2dot*cos(Theta)"
  Square/1 -> Product1/2  "Thetta_dot^2"
  Gain8/1 -> Add2/3  "m * l * Thetta_dot^2 * sin(Thetta)"
  Gain6/1 -> Product2/1, X_dot/1  "x_2dot"
  X/1 -> x/1  "x"
  X_dot/1 -> x_dot/1, Gain2/1, X/1  "x_dot"
  Gain7/1 -> Add2/2  "m * l * Thetta_2dot * cos(Thetta)"
  Product1/1 -> Gain8/1  "Theta_dot^2 * sin(Theta)"
  f/1 -> Add2/1
  Add2/1 -> Gain6/1
  Gain2/1 -> Add2/4

== system Model/Crane 2 ==
  note: Rolling Resistance Model
  f : Inport
  Add2 : Sum  Inputs=+-+-
  Add3 : Sum  Inputs=--
  Cos : Trigonometry  Operator=cos
  Gain10 : Gain  Gain=m*g*L
  Gain2 : Gain  Gain=(m+M)*g*k_cart
  Gain5 : Gain  Gain=1/(m*L^2)
  Gain6 : Gain  Gain=1/(M + m)
  Gain7 : Gain  Gain=m*L
  Gain8 : Gain  Gain=m*L
  Gain9 : Gain  Gain=m*L
  Product : Product
  Product1 : Product
  Product2 : Product
  Sin : Trigonometry
  Square : Math  Operator=square  SaturateOnIntegerOverflow=on
  Theta : Integrator
  Theta_dot : Integrator
  X : Integrator
  X_dot : Integrator
  x : Outport
  x_dot : Outport  Port=2
  theta : Outport  Port=3
  theta_dot : Outport  Port=4
  wires:
  Gain5/1 -> Product/2, Theta_dot/1  "Theta_2dot"
  Gain9/1 -> Add3/1  "m * l * x_2dot*cos(Theta)"
  Add3/1 -> Gain5/1
  Product/1 -> Gain7/1  "Theta_2dot*cos(Thetta)"
  Cos/1 -> Product/1, Product2/2  "cos(Theta)"
  Theta_dot/1 -> theta_dot/1, Square/1, Theta/1  "Theta_dot"
  Sin/1 -> Gain10/1, Product1/1  "sin(Theta)"
  Theta/1 -> theta/1, Cos/1, Sin/1  "Theta"
  Gain10/1 -> Add3/2  "m * g * l * sin(Theta)"
  Product2/1 -> Gain9/1  "x_2dot*cos(Theta)"
  Square/1 -> Product1/2  "Thetta_dot^2"
  Gain8/1 -> Add2/3  "m * l * Thetta_dot^2 * sin(Thetta)"
  Gain6/1 -> Product2/1, X_dot/1  "x_2dot"
  X/1 -> x/1  "x"
  X_dot/1 -> x_dot/1, Gain2/1, X/1  "x_dot"
  Gain7/1 -> Add2/2  "m * l * Thetta_2dot * cos(Thetta)"
  Product1/1 -> Gain8/1  "Theta_dot^2 * sin(Theta)"
  f/1 -> Add2/1
  Add2/1 -> Gain6/1
  Gain2/1 -> Add2/4

== system Model/Crane 3 ==
  note: Rolling Resistance Model
  f : Inport
  Add2 : Sum  Inputs=+-+-
  Add3 : Sum  Inputs=--
  Cos : Trigonometry  Operator=cos
  Gain10 : Gain  Gain=m*g*L
  Gain2 : Gain  Gain=(m+M)*g*k_cart
  Gain5 : Gain  Gain=1/(m*L^2)
  Gain6 : Gain  Gain=1/(M + m)
  Gain7 : Gain  Gain=m*L
  Gain8 : Gain  Gain=m*L
  Gain9 : Gain  Gain=m*L
  Product : Product
  Product1 : Product
  Product2 : Product
  Sin : Trigonometry
  Square : Math  Operator=square  SaturateOnIntegerOverflow=on
  Theta : Integrator
  Theta_dot : Integrator
  X : Integrator
  X_dot : Integrator
  x : Outport
  x_dot : Outport  Port=2
  theta : Outport  Port=3
  theta_dot : Outport  Port=4
  wires:
  Gain5/1 -> Product/2, Theta_dot/1  "Theta_2dot"
  Gain9/1 -> Add3/1  "m * l * x_2dot*cos(Theta)"
  Add3/1 -> Gain5/1
  Product/1 -> Gain7/1  "Theta_2dot*cos(Thetta)"
  Cos/1 -> Product/1, Product2/2  "cos(Theta)"
  Theta_dot/1 -> theta_dot/1, Square/1, Theta/1  "Theta_dot"
  Sin/1 -> Gain10/1, Product1/1  "sin(Theta)"
  Theta/1 -> theta/1, Cos/1, Sin/1  "Theta"
  Gain10/1 -> Add3/2  "m * g * l * sin(Theta)"
  Product2/1 -> Gain9/1  "x_2dot*cos(Theta)"
  Square/1 -> Product1/2  "Thetta_dot^2"
  Gain8/1 -> Add2/3  "m * l * Thetta_dot^2 * sin(Thetta)"
  Gain6/1 -> Product2/1, X_dot/1  "x_2dot"
  X/1 -> x/1  "x"
  X_dot/1 -> x_dot/1, Gain2/1, X/1  "x_dot"
  Gain7/1 -> Add2/2  "m * l * Thetta_2dot * cos(Thetta)"
  Product1/1 -> Gain8/1  "Theta_dot^2 * sin(Theta)"
  f/1 -> Add2/1
  Add2/1 -> Gain6/1
  Gain2/1 -> Add2/4

== system Model/Crane 4 ==
  note: Rolling Resistance Model
  f : Inport
  Add2 : Sum  Inputs=+-+-
  Add3 : Sum  Inputs=--
  Cos : Trigonometry  Operator=cos
  Gain10 : Gain  Gain=m*g*L
  Gain2 : Gain  Gain=(m+M)*g*k_cart
  Gain5 : Gain  Gain=1/(m*L^2)
  Gain6 : Gain  Gain=1/(M + m)
  Gain7 : Gain  Gain=m*L
  Gain8 : Gain  Gain=m*L
  Gain9 : Gain  Gain=m*L
  Product : Product
  Product1 : Product
  Product2 : Product
  Sin : Trigonometry
  Square : Math  Operator=square  SaturateOnIntegerOverflow=on
  Theta : Integrator
  Theta_dot : Integrator
  X : Integrator
  X_dot : Integrator
  x : Outport
  x_dot : Outport  Port=2
  theta : Outport  Port=3
  theta_dot : Outport  Port=4
  wires:
  Gain5/1 -> Product/2, Theta_dot/1  "Theta_2dot"
  Gain9/1 -> Add3/1  "m * l * x_2dot*cos(Theta)"
  Add3/1 -> Gain5/1
  Product/1 -> Gain7/1  "Theta_2dot*cos(Thetta)"
  Cos/1 -> Product/1, Product2/2  "cos(Theta)"
  Theta_dot/1 -> theta_dot/1, Square/1, Theta/1  "Theta_dot"
  Sin/1 -> Gain10/1, Product1/1  "sin(Theta)"
  Theta/1 -> theta/1, Cos/1, Sin/1  "Theta"
  Gain10/1 -> Add3/2  "m * g * l * sin(Theta)"
  Product2/1 -> Gain9/1  "x_2dot*cos(Theta)"
  Square/1 -> Product1/2  "Thetta_dot^2"
  Gain8/1 -> Add2/3  "m * l * Thetta_dot^2 * sin(Thetta)"
  Gain6/1 -> Product2/1, X_dot/1  "x_2dot"
  X/1 -> x/1  "x"
  X_dot/1 -> x_dot/1, Gain2/1, X/1  "x_dot"
  Gain7/1 -> Add2/2  "m * l * Thetta_2dot * cos(Thetta)"
  Product1/1 -> Gain8/1  "Theta_dot^2 * sin(Theta)"
  f/1 -> Add2/1
  Add2/1 -> Gain6/1
  Gain2/1 -> Add2/4
